simulink model "lab_007_sim2015"  (R2016a)
settings: Solver=ode8  SolverMode=SingleTasking  StartTime=0.0  StopTime=20.0  FixedStep=1e-2  RelTol=1e-3
values from neighbouring files (symbols this model uses):
  C = C + c1    (= 0.1)    [lab7_checkResults.m]    (also in lab7_prepareData.m = 0.2; lab_007.m = 0.2)
  K = K + k1    (= 0.1)    [lab7_checkResults.m]    (also in lab7_prepareData.m = 0.2; lab_007.m = 0.2)
  m = 2    [lab7_prepareData.m]    (also in lab_007.m)
settings Model: Creator=kamzab95  LastModifiedBy=Bartek
settings DebuggingCC: SFUnexpectedBacktrackingDiag=error  SFNoUnconditionalDefaultTransitionDiag=error
settings HardwareCC: ProdWordSize=32  ProdHWDeviceType=Specified
settings GRTTargetCC: TargetLangStandard=C99 (ISO)  GeneratePreprocessorConditionals=Use local settings
settings ConfigComp: CovMetricSettings=dwe  CovHtmlReporting=off  CovSaveCumulativeToWorkspaceVar=off  CovSaveSingleToWorkspaceVar=off  CovModelRefEnable=Off  CovExternalEMLEnable=on

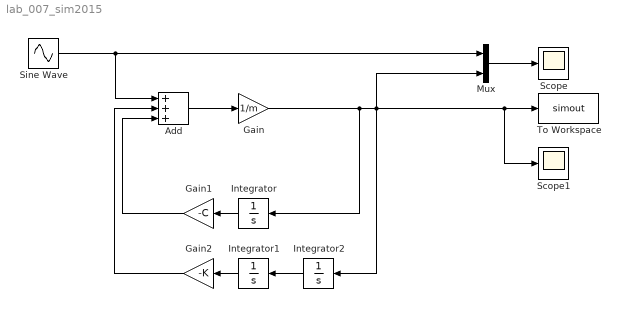
== system lab_007_sim2015 ==
  Add : Sum  Inputs=+++
  Gain : Gain  Gain=1/m
  Gain1 : Gain  Gain=-C
  Gain2 : Gain  Gain=-K
  Integrator : Integrator
  Integrator1 : Integrator
  Integrator2 : Integrator
  Mux : Mux  Inputs=2
  Scope : Scope
  Scope1 : Scope
  Sine Wave : Sin  SampleTime=0
  To Workspace : ToWorkspace  VariableName=simout  SaveFormat=Timeseries  SampleTime=-1
  wires:
  Sine Wave/1 -> Mux/1, Add/1
  Gain/1 -> Integrator/1, Integrator2/1, Scope1/1, To Workspace/1, Mux/2
  Add/1 -> Gain/1
  Mux/1 -> Scope/1
  Integrator1/1 -> Gain2/1
  Integrator/1 -> Gain1/1
  Gain2/1 -> Add/2
  Gain1/1 -> Add/3
  Integrator2/1 -> Integrator1/1
